simulink model "p1_MPU"  (R2023a)
settings: Solver=FixedStepDiscrete  StartTime=0.0  StopTime=inf  FixedStep=Ts_MPU  RelTol=1e-3  EnableMultiTasking=on
PreLoadFcn:
  | p1_params_new
  | spiDataDefinition
InitFcn:
  | p1_params_new
  | spiDataDefinition
values from neighbouring files (symbols this model uses):
  B = SSest(T,15)+Boffset    [AACplottingcode.m]    (also in Ext_MPCPara.m = SSD.B; IMECE06plottingcode.m = SSest(T,15); If_alpha_tp_observer.m; If_alpha_tp_observer_for_c_code.m)
undefined symbols (not defined in the file or in its folder): DrivetrainLeft, DrivetrainRight, p1data, p1params, Ts_MPU
libraries: simulink x54, raspberrypiBasiclib x8, raspberrypiCommlib x4, embedlinuxNetworklib x2
(part 1 of 2)
settings Model: SimulationMode=external  ExtModeTrigDuration=2  Creator=Audesse  LastModifiedBy=cbeal
settings SolverCC: AlgebraicLoopSolver=TrustRegion  PositivePriorityOrder=on
settings DataIOCC: ReturnWorkspaceOutputs=off  LoggingFileName=MPU_Data.mat
settings OptimizationCC: DefaultUnderspecifiedDataType=single  EnhancedBackFolding=on  PassReuseOutputArgsAs=Individual arguments  MaxStackSize=64  SimCompilerOptimization=on  OptimizeBlockOrder=speed  DifferentSizesBufferReuse=on  OptimizationCustomize=off  EfficientTunableParamExpr=on
settings DebuggingCC: MultiTaskDSMMsg=none  ParameterTunabilityLossMsg=error  UnconnectedInputMsg=warning  UnconnectedOutputMsg=warning  UnconnectedLineMsg=warning
settings HardwareCC: ProdBitPerPointer=32  ProdBitPerSizeT=32  ProdBitPerPtrDiffT=32  ProdLargestAtomicInteger=Long  ProdLargestAtomicFloat=Double  ProdWordSize=32  ProdLongLongMode=on  ProdHWDeviceType=ARM Compatible->ARM Cortex  TargetLargestAtomicInteger=Long  TargetLargestAtomicFloat=Double  TargetLongLongMode=on  TargetIntDivRoundTo=Zero  TargetEndianess=LittleEndian  TargetHWDeviceType=ARM Compatible->ARM Cortex
settings ModelReferenceCC: EnableRefExpFcnMdlSchedulingChecks=on
settings SFSimCC: CustomCodeUndefinedFunction=UseInterfaceOnly
settings RTWCC: Description=Embedded Coder  SystemTargetFile=ert.tlc  HardwareBoard=Raspberry Pi  TLCOptions="-aInlineSetEventsForThisBaseRateFcn=TLC_FALSE -aSuppressMultiTaskScheduler=TLC_FALSE  -aRateBasedStepFcn=0"  TemplateMakefile=ert_default_tmf  Toolchain=GNU GCC Embedded Linux  BuildConfiguration=Faster Runs  IncludeHyperlinkInReport=on  CodeExecutionProfiling=on  CodeProfilingSaveOptions=AllData  CodeProfilingInstrumentation=coarse  DLArmComputeVersion=19.05
settings CodeAppCC: ForceParamTrailComments=on  IgnoreCustomStorageClasses=off  OperatorAnnotations=on  SimulinkDataObjDesc=on  SFDataObjDesc=on  MangleLength=10  InsertBlockDesc=on
settings ERTTargetCC: MatFileLogging=on  SupportNonInlinedSFcns=on  SupportVariableSizeSignals=on  ExtModeTransport=2  ExtModeStaticAlloc=on  ExtModeMexFile=ext_xcp  ExtModeIntrfLevel=Level2 - Open

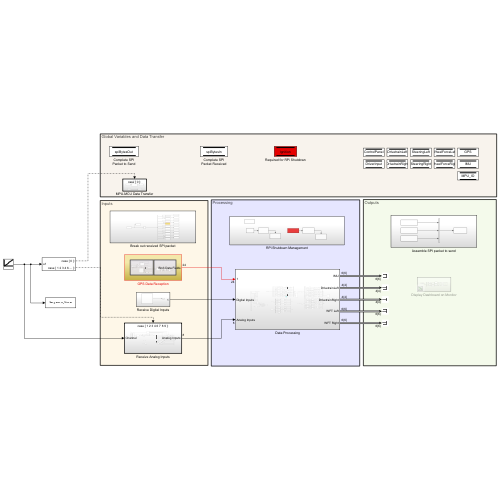
[thumbnail: Simulink's stored preview of the top-level diagram]
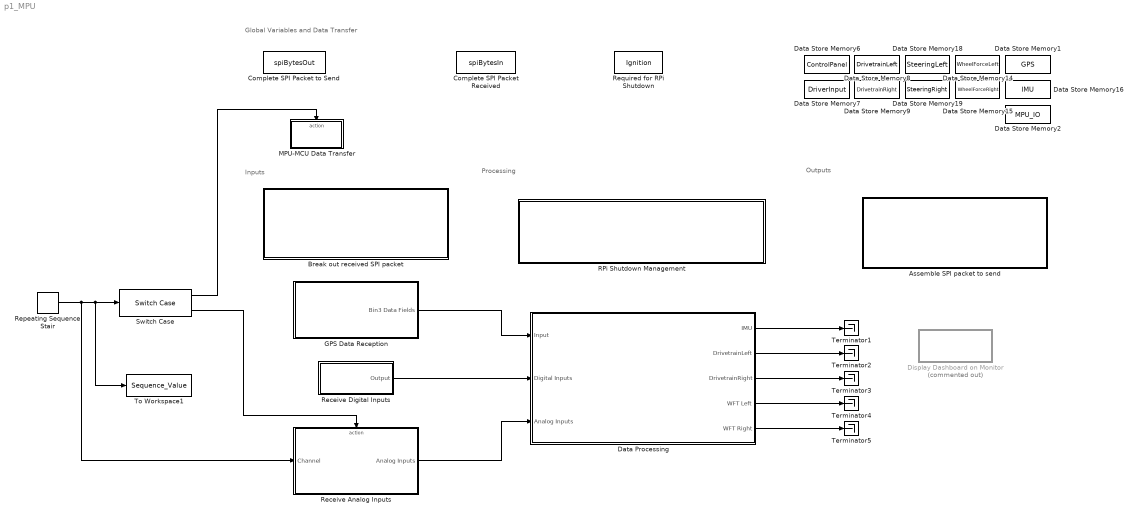
== system p1_MPU ==
  note: Outputs
  note: Processing
  note: Inputs
  note: Global Variables and Data Transfer
  Assemble SPI packet to send : Subsystem
  Break out received SPI packet : Subsystem
  Complete SPI Packet Received : DataStoreMemory  DataStoreName=spiBytesIn  ReadBeforeWriteMsg=warning  WriteAfterWriteMsg=warning  WriteAfterReadMsg=warning  InitialValue=255*ones(p1data.spiBytes,1)  ShowAdditionalParam=off  OutDataTypeStr=uint8
  Complete SPI Packet to Send : DataStoreMemory  DataStoreName=spiBytesOut  ReadBeforeWriteMsg=warning  WriteAfterWriteMsg=warning  WriteAfterReadMsg=warning  InitialValue=zeros(p1data.spiBytes,1)  ShowAdditionalParam=off  OutDataTypeStr=uint8
  Data Processing : Subsystem
  Data Store Memory1 : DataStoreMemory  DataStoreName=GPS  ReadBeforeWriteMsg=warning  WriteAfterWriteMsg=warning  WriteAfterReadMsg=warning  InitialValue=zeros(p1data.gpsBytes,1)  ShowAdditionalParam=off  OutDataTypeStr=uint8
  Data Store Memory14 : DataStoreMemory  DataStoreName=WheelForceLeft  ReadBeforeWriteMsg=warning  WriteAfterWriteMsg=warning  WriteAfterReadMsg=warning  InitialValue=zeros(p1data.wftBytes,1)  ShowAdditionalParam=off  OutDataTypeStr=uint8
  Data Store Memory15 : DataStoreMemory  DataStoreName=WheelForceRight  ReadBeforeWriteMsg=warning  WriteAfterWriteMsg=warning  WriteAfterReadMsg=warning  InitialValue=zeros(p1data.wftBytes,1)  ShowAdditionalParam=off  OutDataTypeStr=uint8
  Data Store Memory16 : DataStoreMemory  DataStoreName=IMU  ReadBeforeWriteMsg=warning  WriteAfterWriteMsg=warning  WriteAfterReadMsg=warning  InitialValue=zeros(p1data.imuBytes,1)  ShowAdditionalParam=off  OutDataTypeStr=uint8
  Data Store Memory18 : DataStoreMemory  DataStoreName=SteeringLeft  ReadBeforeWriteMsg=warning  WriteAfterWriteMsg=warning  WriteAfterReadMsg=warning  InitialValue=zeros(p1data.steeringBytes,1)  ShowAdditionalParam=off  OutDataTypeStr=uint8
  Data Store Memory19 : DataStoreMemory  DataStoreName=SteeringRight  ReadBeforeWriteMsg=warning  WriteAfterWriteMsg=warning  WriteAfterReadMsg=warning  InitialValue=zeros(p1data.steeringBytes,1)  ShowAdditionalParam=off  OutDataTypeStr=uint8
  Data Store Memory2 : DataStoreMemory  DataStoreName=MPU_IO  ReadBeforeWriteMsg=warning  WriteAfterWriteMsg=warning  WriteAfterReadMsg=warning  InitialValue=zeros(p1data.mpuBytes,1)  ShowAdditionalParam=off  OutDataTypeStr=uint8
  Data Store Memory6 : DataStoreMemory  DataStoreName=ControlPanel  ReadBeforeWriteMsg=warning  WriteAfterWriteMsg=warning  WriteAfterReadMsg=warning  InitialValue=zeros(p1data.controlPanelBytes,1)  ShowAdditionalParam=off  OutDataTypeStr=uint8
  Data Store Memory7 : DataStoreMemory  DataStoreName=DriverInput  ReadBeforeWriteMsg=warning  WriteAfterWriteMsg=warning  WriteAfterReadMsg=warning  InitialValue=zeros(p1data.driverInputBytes,1)  ShowAdditionalParam=off  OutDataTypeStr=uint8
  Data Store Memory8 : DataStoreMemory  DataStoreName=DrivetrainLeft  ReadBeforeWriteMsg=warning  WriteAfterWriteMsg=warning  WriteAfterReadMsg=warning  InitialValue=zeros(p1data.drivetrainBytes,1)  ShowAdditionalParam=off  OutDataTypeStr=uint8
  Data Store Memory9 : DataStoreMemory  DataStoreName=DrivetrainRight  ReadBeforeWriteMsg=warning  WriteAfterWriteMsg=warning  WriteAfterReadMsg=warning  InitialValue=zeros(p1data.drivetrainBytes,1)  ShowAdditionalParam=off  OutDataTypeStr=uint8
  Display Dashboard on Monitor : Subsystem  Commented=on
  GPS Data Reception : Subsystem
  MPU-MCU Data Transfer : Subsystem  TreatAsAtomicUnit=on
  RPi Shutdown Management : Subsystem
  Receive Analog Inputs : Subsystem  TreatAsAtomicUnit=on
  Receive Digital Inputs : Subsystem
  Repeating Sequence Stair : simulink/Sources/Repeating Sequence Stair  OutValues=(0:9)'  tsamp=-1  OutMin=[]  OutMax=[]  OutDataTypeStr=uint8  OutputDataTypeScalingMode=uint8  OutDataType=fixdt(0,8)  ConRadixGroup=Best Precision: Vector-wise  OutScaling=2^-12
  Required for RPi Shutdown : DataStoreMemory  DataStoreName=Ignition  ReadBeforeWriteMsg=warning  WriteAfterWriteMsg=warning  WriteAfterReadMsg=warning  ShowAdditionalParam=off  OutDataTypeStr=uint8
  Switch Case : SwitchCase  CaseConditions={[0],[1,2,3,4,6,7,8,9]}  ShowDefaultCase=off
  Terminator{1..5} (5 alike) : Terminator
  To Workspace1 : ToWorkspace  VariableName=Sequence_Value  SampleTime=-1
  wires:
  Data Processing/1(IMU) -> Terminator1/1
  Data Processing/2(DrivetrainLeft) -> Terminator2/1
  Data Processing/3(DrivetrainRight) -> Terminator3/1
  Data Processing/4(WFT Left) -> Terminator4/1
  Data Processing/5(WFT Right) -> Terminator5/1
  Switch Case/1 -> MPU-MCU Data Transfer/Action
  Receive Analog Inputs/1(Analog Inputs) -> Data Processing/3(Analog Inputs)
  Receive Digital Inputs/1(Output) -> Data Processing/2(Digital Inputs)
  GPS Data Reception/1(Bin3 Data Fields) -> Data Processing/1(Input)
  Repeating Sequence Stair/1 -> Switch Case/1, To Workspace1/1, Receive Analog Inputs/1(Channel)
  Switch Case/2 -> Receive Analog Inputs/Action

== system p1_MPU/Assemble SPI packet to send ==
  Data Store Read : DataStoreRead  DataStoreName=GPS  IndexOptions=Index vector (dialog)  Indices=1  OutputSizes=1
  Data Store Read1 : DataStoreRead  DataStoreName=MPU_IO  IndexOptions=Index vector (dialog)  Indices=1  OutputSizes=1
  Data Store Write : DataStoreWrite  DataStoreName=spiBytesOut  IndexOptions=Index vector (dialog)  Indices=1  OutputSizes=1
  Mux : Mux  Inputs=3
  Padding : Constant  Value=zeros(p1data.mpuPadding,1)  OutDataTypeStr=uint8
  wires:
  Mux/1 -> Data Store Write/1
  Padding/1 -> Mux/3
  Data Store Read/1 -> Mux/1
  Data Store Read1/1 -> Mux/2

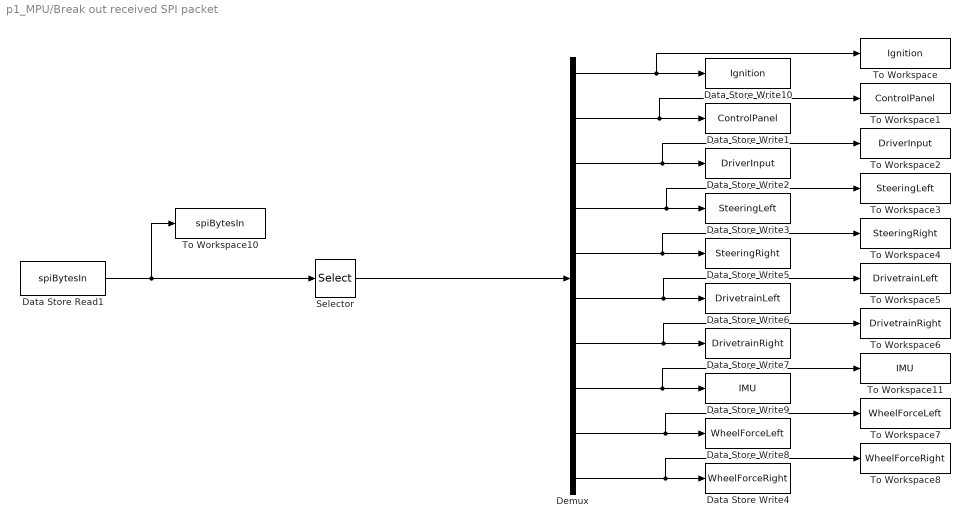
== system p1_MPU/Break out received SPI packet ==
  Data Store Read1 : DataStoreRead  DataStoreName=spiBytesIn  IndexOptions=Index vector (dialog)  Indices=1  OutputSizes=1
  Data Store Write1 : DataStoreWrite  DataStoreName=ControlPanel  IndexOptions=Index vector (dialog)  Indices=1  OutputSizes=1
  Data Store Write10 : DataStoreWrite  DataStoreName=Ignition  IndexOptions=Index vector (dialog)  Indices=1  OutputSizes=1
  Data Store Write2 : DataStoreWrite  DataStoreName=DriverInput  IndexOptions=Index vector (dialog)  Indices=1  OutputSizes=1
  Data Store Write3 : DataStoreWrite  DataStoreName=SteeringLeft  IndexOptions=Index vector (dialog)  Indices=1  OutputSizes=1
  Data Store Write4 : DataStoreWrite  DataStoreName=WheelForceRight  IndexOptions=Index vector (dialog)  Indices=1  OutputSizes=1
  Data Store Write5 : DataStoreWrite  DataStoreName=SteeringRight  IndexOptions=Index vector (dialog)  Indices=1  OutputSizes=1
  Data Store Write6 : DataStoreWrite  DataStoreName=DrivetrainLeft  IndexOptions=Index vector (dialog)  Indices=1  OutputSizes=1
  Data Store Write7 : DataStoreWrite  DataStoreName=DrivetrainRight  IndexOptions=Index vector (dialog)  Indices=1  OutputSizes=1
  Data Store Write8 : DataStoreWrite  DataStoreName=WheelForceLeft  IndexOptions=Index vector (dialog)  Indices=1  OutputSizes=1
  Data Store Write9 : DataStoreWrite  DataStoreName=IMU  IndexOptions=Index vector (dialog)  Indices=1  OutputSizes=1
  Demux : Demux  Outputs=10
  Selector : Selector  InputPortWidth=p1data.spiBytes  IndexOptions=Index vector (dialog)  Indices=[11:225]  OutputSizes=1
  To Workspace : ToWorkspace  VariableName=Ignition  SampleTime=-1
  To Workspace1 : ToWorkspace  VariableName=ControlPanel  SampleTime=-1
  To Workspace10 : ToWorkspace  VariableName=spiBytesIn  SampleTime=-1
      settings: Save2DSignal=2-D array (concatenate along first dimension)
  To Workspace11 : ToWorkspace  VariableName=IMU  SampleTime=-1
  To Workspace2 : ToWorkspace  VariableName=DriverInput  SampleTime=-1
  To Workspace3 : ToWorkspace  VariableName=SteeringLeft  SampleTime=-1
  To Workspace4 : ToWorkspace  VariableName=SteeringRight  SampleTime=-1
  To Workspace5 : ToWorkspace  VariableName=DrivetrainLeft  SampleTime=-1
  To Workspace6 : ToWorkspace  VariableName=DrivetrainRight  SampleTime=-1
  To Workspace7 : ToWorkspace  VariableName=WheelForceLeft  SampleTime=-1
  To Workspace8 : ToWorkspace  VariableName=WheelForceRight  SampleTime=-1
  wires:
  Demux/5 -> Data Store Write5/1, To Workspace4/1
  Demux/1 -> To Workspace/1, Data Store Write10/1
  Demux/9 -> To Workspace7/1, Data Store Write8/1
  Demux/4 -> To Workspace3/1, Data Store Write3/1
  Demux/2 -> Data Store Write1/1, To Workspace1/1
  Demux/6 -> To Workspace5/1, Data Store Write6/1
  Demux/7 -> To Workspace6/1, Data Store Write7/1
  Demux/3 -> To Workspace2/1, Data Store Write2/1
  Demux/10 -> To Workspace8/1, Data Store Write4/1
  Demux/8 -> To Workspace11/1, Data Store Write9/1
  Data Store Read1/1 -> Selector/1, To Workspace10/1
  Selector/1 -> Demux/1

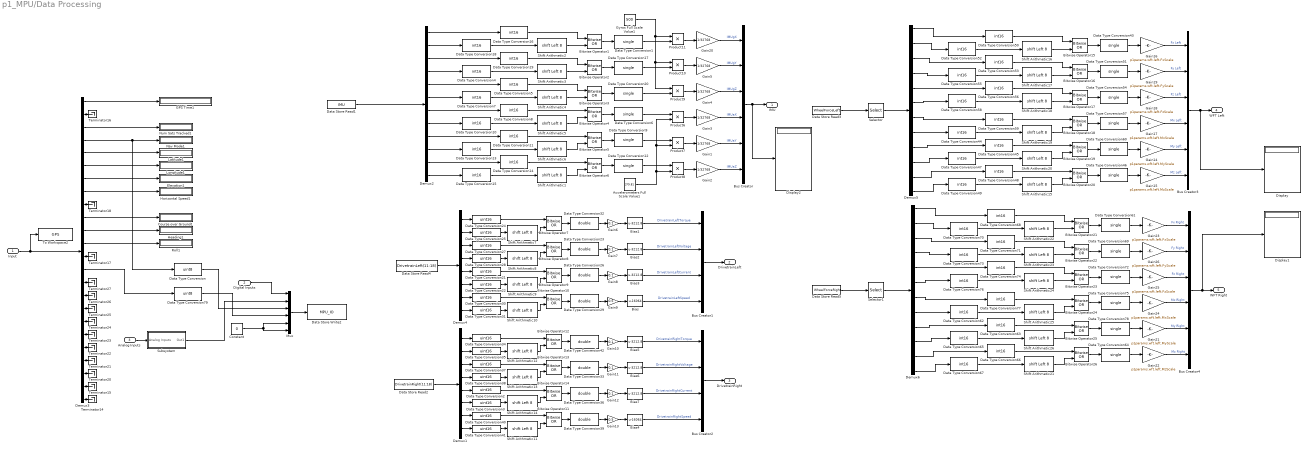
== system p1_MPU/Data Processing ==
  Input : Inport
  Digital Inputs : Inport  Port=2
  Analog Inputs : Inport  Port=3
  Accelerometers Full Scale Value1 : Constant  Value=2*9.81
  Bias : Bias  Bias=-16064  SaturateOnIntegerOverflow=off
  Bias{1..3,5..7} (6 alike) : Bias  Bias=-3212.8  SaturateOnIntegerOverflow=off
  Bias4 : Bias  Bias=-16064  SaturateOnIntegerOverflow=off
  Bitwise Operator{1..26} (26 alike) : simulink/Logic and Bit Operations/Bitwise Operator  logicop=OR  UseBitMask=off  NumInputPorts=2  BitMask=bin2dec('11011001')  BitMaskRealWorld=Stored Integer
  Bus Creator : BusCreator  Inputs=6
  Bus Creator1 : BusCreator  Inputs=4
  Bus Creator2 : BusCreator  Inputs=4
  Bus Creator3 : BusCreator  Inputs=6
  Bus Creator4 : BusCreator  Inputs=6
  Constant : Constant  Value=0  OutDataTypeStr=uint8
  Course over Ground1 : Display
  Data Store Read1 : DataStoreRead  DataStoreName=IMU  IndexOptions=Index vector (dialog)  Indices=1  OutputSizes=1
  Data Store Read2 : DataStoreRead  DataStoreName=DrivetrainRight  DataStoreElements=DrivetrainRight(11:18)  IndexOptions=Index vector (dialog)  Indices=1  OutputSizes=1
  Data Store Read3 : DataStoreRead  DataStoreName=WheelForceLeft  IndexOptions=Index vector (dialog)  Indices=1  OutputSizes=1
  Data Store Read4 : DataStoreRead  DataStoreName=DrivetrainLeft  DataStoreElements=DrivetrainLeft(11:18)  IndexOptions=Index vector (dialog)  Indices=1  OutputSizes=1
  Data Store Read5 : DataStoreRead  DataStoreName=WheelForceRight  IndexOptions=Index vector (dialog)  Indices=1  OutputSizes=1
  Data Store Write2 : DataStoreWrite  DataStoreName=MPU_IO  IndexOptions=Index vector (dialog)  Indices=1  OutputSizes=1
  Data Type Conversion : DataTypeConversion  OutDataTypeStr=uint8  SaturateOnIntegerOverflow=off  RndMeth=Floor
  Data Type Conversion{1,6,9,12,17,20,43,46,51,54,57,60..61,64,69,72,75,78} (18 alike) : DataTypeConversion  OutDataTypeStr=single  SaturateOnIntegerOverflow=off  RndMeth=Floor
  Data Type Conversion{4..5,7..8,10..11,13..16,18..19,44..45,47..50,52..53,55..56,58..59,62..63,65..68,70..71,73..74,76..77} (36 alike) : DataTypeConversion  OutDataTypeStr=int16  ConvertRealWorld=Stored Integer (SI)  SaturateOnIntegerOverflow=off  RndMeth=Floor
  Data Type Conversion{2..3,21..22,24..25,27..28,30..31,34..35,37..38,40..41} (16 alike) : DataTypeConversion  OutDataTypeStr=uint16  SaturateOnIntegerOverflow=off  RndMeth=Floor
  Data Type Conversion{23,26,29,32..33,36,39,42} (8 alike) : DataTypeConversion  OutDataTypeStr=double  SaturateOnIntegerOverflow=off  RndMeth=Floor
  Data Type Conversion79 : DataTypeConversion  OutDataTypeStr=uint8  SaturateOnIntegerOverflow=off  RndMeth=Floor
  Demux1 : Demux  Outputs=8
  Demux2 : Demux  Outputs=12
  Demux3 : Demux  Outputs=24
  Demux4 : Demux  Outputs=8
  Demux5 : Demux  Outputs=12
  Demux6 : Demux  Outputs=12
  Display : Display
  Display1 : Display
  Display2 : Display
  Elevation1 : Display
  GPS Time1 : Display
      settings: Format=long_e
  Gain{1..5,20} (6 alike) : Gain  Gain=1/32768
  Gain{6..8,10..12} (6 alike) : Gain  Gain=0.1  OutDataTypeStr=Inherit: Same as input
  Gain13 : Gain  Gain=0.5  OutDataTypeStr=Inherit: Same as input
  Gain14 : Gain  Gain=p1params.wft.left.MyScale
  Gain15 : Gain  Gain=p1params.wft.left.MzScale
  Gain16 : Gain  Gain=p1params.wft.left.FxScale
  Gain17 : Gain  Gain=p1params.wft.left.MxScale
  Gain18 : Gain  Gain=p1params.wft.left.FzScale
  Gain19 : Gain  Gain=p1params.wft.left.FyScale
  Gain21 : Gain  Gain=p1params.wft.left.MyScale
  Gain22 : Gain  Gain=p1params.wft.left.MzScale
  Gain23 : Gain  Gain=p1params.wft.left.FxScale
  Gain24 : Gain  Gain=p1params.wft.left.MxScale
  Gain25 : Gain  Gain=p1params.wft.left.FzScale
  Gain26 : Gain  Gain=p1params.wft.left.FyScale
  Gain9 : Gain  Gain=0.5  OutDataTypeStr=Inherit: Same as input
  Gyros Full Scale Value1 : Constant  Value=500
  Heading1 : Display
  Horizontal Speed1 : Display
  Latitude1 : Display
  Longitude1 : Display
  Mux : Mux  Inputs=6
  Nav Mode1 : Display
  Num Sats Tracked1 : Display
  Product{6..11} (6 alike) : Product
  Roll1 : Display
  Selector : Selector  InputPortWidth=20  IndexOptions=Index vector (dialog)  Indices=[1:12]  OutputSizes=1
  Selector1 : Selector  InputPortWidth=20  IndexOptions=Index vector (dialog)  Indices=[1:12]  OutputSizes=1
  Shift Arithmetic{1..26} (26 alike) : ArithShift  BitShiftNumber=8  BitShiftDirection=Left
  Subsystem : Subsystem
  Terminator{14..18,20..27} (13 alike) : Terminator
  To Workspace2 : ToWorkspace  VariableName=GPS  SampleTime=-1
      settings: Save2DSignal=2-D array (concatenate along first dimension)
  IMU : Outport
  DrivetrainLeft : Outport  Port=2
  DrivetrainRight : Outport  Port=3
  WFT Left : Outport  Port=4
  WFT Right : Outport  Port=5
  wires:
  Data Store Read1/1 -> Demux2/1
  Data Type Conversion23/1 -> Gain7/1
  Data Type Conversion26/1 -> Gain8/1
  Data Type Conversion32/1 -> Gain6/1
  Demux4/8 -> Data Type Conversion31/1
  Data Type Conversion30/1 -> Bitwise Operator10/1
  Gain6/1 -> Bias1/1
  Data Type Conversion29/1 -> Gain9/1
  Demux4/7 -> Data Type Conversion30/1
  Bitwise Operator10/1 -> Data Type Conversion29/1
  Bitwise Operator7/1 -> Data Type Conversion32/1
  Bitwise Operator9/1 -> Data Type Conversion26/1
  Bitwise Operator8/1 -> Data Type Conversion23/1
  Data Store Read4/1 -> Demux4/1
  Demux4/1 -> Data Type Conversion24/1
  Demux4/2 -> Data Type Conversion25/1
  Demux4/3 -> Data Type Conversion27/1
  Demux4/4 -> Data Type Conversion28/1
  Demux4/5 -> Data Type Conversion21/1
  Demux4/6 -> Data Type Conversion22/1
  Data Type Conversion21/1 -> Bitwise Operator9/1
  Data Type Conversion27/1 -> Bitwise Operator8/1
  Data Type Conversion24/1 -> Bitwise Operator7/1
  Bias1/1 -> Bus Creator1/1  "DrivetrainLeftTorque"
  Gain7/1 -> Bias2/1
  Bias2/1 -> Bus Creator1/2  "DrivetrainLeftVoltage"
  Gain9/1 -> Bias/1
  Bias/1 -> Bus Creator1/4  "DrivetrainLeftSpeed"
  Gain8/1 -> Bias3/1
  Bias3/1 -> Bus Creator1/3  "DrivetrainLeftCurrent"
  Data Type Conversion25/1 -> Shift Arithmetic7/1
  Data Type Conversion31/1 -> Shift Arithmetic10/1
  Data Type Conversion22/1 -> Shift Arithmetic9/1
  Data Type Conversion28/1 -> Shift Arithmetic8/1
  Shift Arithmetic7/1 -> Bitwise Operator7/2
  Shift Arithmetic8/1 -> Bitwise Operator8/2
  Shift Arithmetic9/1 -> Bitwise Operator9/2
  Shift Arithmetic10/1 -> Bitwise Operator10/2
  Shift Arithmetic11/1 -> Bitwise Operator11/2
  Shift Arithmetic14/1 -> Bitwise Operator14/2
  Shift Arithmetic13/1 -> Bitwise Operator13/2
  Shift Arithmetic12/1 -> Bitwise Operator12/2
  Data Type Conversion38/1 -> Shift Arithmetic13/1
  Data Type Conversion3/1 -> Shift Arithmetic14/1
  Data Type Conversion41/1 -> Shift Arithmetic11/1
  Data Type Conversion35/1 -> Shift Arithmetic12/1
  Gain12/1 -> Bias7/1
  Gain13/1 -> Bias4/1
  Gain11/1 -> Bias6/1
  Data Type Conversion34/1 -> Bitwise Operator12/1
  Data Type Conversion37/1 -> Bitwise Operator13/1
  Data Type Conversion2/1 -> Bitwise Operator14/1
  Demux1/6 -> Data Type Conversion3/1
  Demux1/5 -> Data Type Conversion2/1
  Demux1/4 -> Data Type Conversion38/1
  Demux1/3 -> Data Type Conversion37/1
  Demux1/2 -> Data Type Conversion35/1
  Demux1/1 -> Data Type Conversion34/1
  Data Store Read2/1 -> Demux1/1
  Bitwise Operator13/1 -> Data Type Conversion33/1
  Bitwise Operator14/1 -> Data Type Conversion36/1
  Bitwise Operator12/1 -> Data Type Conversion42/1
  Bitwise Operator11/1 -> Data Type Conversion39/1
  Demux1/7 -> Data Type Conversion40/1
  Data Type Conversion39/1 -> Gain13/1
  Gain10/1 -> Bias5/1
  Data Type Conversion40/1 -> Bitwise Operator11/1
  Demux1/8 -> Data Type Conversion41/1
  Data Type Conversion42/1 -> Gain10/1
  Data Type Conversion36/1 -> Gain12/1
  Data Type Conversion33/1 -> Gain11/1
  Bus Creator/1 -> Display2/1, IMU/1
  Bias5/1 -> Bus Creator2/1  "DrivetrainRightTorque"
  Bias6/1 -> Bus Creator2/2  "DrivetrainRightVoltage"
  Bias4/1 -> Bus Creator2/4  "DrivetrainRightSpeed"
  Bias7/1 -> Bus Creator2/3  "DrivetrainRightCurrent"
  Bus Creator1/1 -> DrivetrainLeft/1
  Bus Creator2/1 -> DrivetrainRight/1
  Gyros Full Scale Value1/1 -> Product9/1, Product10/1, Product11/1
  Data Type Conversion10/1 -> Shift Arithmetic5/1
  Data Type Conversion17/1 -> Product10/2
  Demux2/9 -> Data Type Conversion11/1
  Bitwise Operator6/1 -> Data Type Conversion12/1
  Demux2/6 -> Data Type Conversion7/1
  Data Type Conversion20/1 -> Product9/2
  Data Type Conversion13/1 -> Shift Arithmetic6/1
  Product11/1 -> Gain20/1
  Product10/1 -> Gain5/1
  Accelerometers Full Scale Value1/1 -> Product6/2, Product7/2, Product8/2
  Demux2/2 -> Data Type Conversion18/1
  Data Type Conversion6/1 -> Product6/1
  Demux2/1 -> Data Type Conversion16/1
  Bitwise Operator1/1 -> Data Type Conversion1/1
  Data Type Conversion15/1 -> Shift Arithmetic1/1
  Bitwise Operator4/1 -> Data Type Conversion6/1
  Product7/1 -> Gain1/1
  Shift Arithmetic5/1 -> Bitwise Operator4/2
  Product9/1 -> Gain4/1
  Product8/1 -> Gain2/1
  Data Type Conversion19/1 -> Bitwise Operator2/1
  Data Type Conversion9/1 -> Product7/1
  Data Type Conversion4/1 -> Shift Arithmetic3/1
  Data Type Conversion12/1 -> Product8/1
  Shift Arithmetic3/1 -> Bitwise Operator2/2
  Bitwise Operator3/1 -> Data Type Conversion20/1
  Product6/1 -> Gain3/1
  Bitwise Operator2/1 -> Data Type Conversion17/1
  Data Type Conversion1/1 -> Product11/2
  Data Type Conversion7/1 -> Shift Arithmetic4/1
  Shift Arithmetic2/1 -> Bitwise Operator1/2
  Data Type Conversion18/1 -> Shift Arithmetic2/1
  Shift Arithmetic4/1 -> Bitwise Operator3/2
  Demux2/4 -> Data Type Conversion4/1
  Shift Arithmetic6/1 -> Bitwise Operator5/2
  Demux2/10 -> Data Type Conversion13/1
  Bitwise Operator5/1 -> Data Type Conversion9/1
  Demux2/3 -> Data Type Conversion19/1
  Shift Arithmetic1/1 -> Bitwise Operator6/2
  Data Type Conversion16/1 -> Bitwise Operator1/1
  Data Type Conversion5/1 -> Bitwise Operator3/1
  Data Type Conversion14/1 -> Bitwise Operator6/1
  Data Type Conversion8/1 -> Bitwise Operator4/1
  Demux2/5 -> Data Type Conversion5/1
  Demux2/8 -> Data Type Conversion10/1
  Data Type Conversion11/1 -> Bitwise Operator5/1
  Demux2/7 -> Data Type Conversion8/1
  Demux2/12 -> Data Type Conversion15/1
  Demux2/11 -> Data Type Conversion14/1
  Gain2/1 -> Bus Creator/6  "IMUaZ"
  Gain1/1 -> Bus Creator/5  "IMUaY"
  Gain3/1 -> Bus Creator/4  "IMUaX"
  Gain4/1 -> Bus Creator/3  "IMUgZ"
  Gain5/1 -> Bus Creator/2  "IMUgY"
  Gain20/1 -> Bus Creator/1  "IMUgX"
  Demux3/5 -> Latitude1/1
  Demux3/8 -> Horizontal Speed1/1
  Demux3/7 -> Elevation1/1
  Demux3/22 -> Terminator20/1
  Demux3/11 -> Heading1/1
  Demux3/6 -> Longitude1/1
  Demux3/1 -> GPS Time1/1
  Demux3/3 -> Num Sats Tracked1/1
  Demux3/21 -> Terminator21/1
  Demux3/20 -> Terminator22/1
  Demux3/9 -> Terminator18/1
  Demux3/15 -> Terminator27/1
  Demux3/19 -> Terminator23/1
  Demux3/24 -> Terminator14/1
  Demux3/10 -> Course over Ground1/1
  Demux3/17 -> Terminator25/1
  Demux3/12 -> Roll1/1
  Demux3/16 -> Terminator26/1
  Demux3/13 -> Terminator17/1
  Demux3/18 -> Terminator24/1
  Demux3/23 -> Terminator15/1
  Demux3/2 -> Terminator16/1
  Input/1 -> Demux3/1, To Workspace2/1
  Shift Arithmetic16/1 -> Bitwise Operator15/2
  Shift Arithmetic17/1 -> Bitwise Operator16/2
  Data Type Conversion45/1 -> Bitwise Operator19/1
  Data Type Conversion56/1 -> Bitwise Operator17/1
  Data Type Conversion57/1 -> Gain17/1
  Bitwise Operator16/1 -> Data Type Conversion51/1
  Shift Arithmetic20/1 -> Bitwise Operator19/2
  Gain14/1 -> Bus Creator3/5  "My Left"
  Demux5/6 -> Data Type Conversion58/1
  Data Type Conversion58/1 -> Shift Arithmetic18/1
  Data Type Conversion55/1 -> Shift Arithmetic17/1
  Data Type Conversion50/1 -> Bitwise Operator15/1
  Demux5/11 -> Data Type Conversion48/1
  Shift Arithmetic19/1 -> Bitwise Operator18/2
  Bitwise Operator18/1 -> Data Type Conversion57/1
  Demux5/8 -> Data Type Conversion44/1
  Demux5/3 -> Data Type Conversion53/1
  Data Type Conversion52/1 -> Shift Arithmetic16/1
  Demux5/4 -> Data Type Conversion55/1
  Gain15/1 -> Bus Creator3/6  "Mz Left"
  Demux5/7 -> Data Type Conversion59/1
  Demux5/10 -> Data Type Conversion47/1
  Bitwise Operator19/1 -> Data Type Conversion60/1
  Data Type Conversion47/1 -> Shift Arithmetic20/1
  Demux5/2 -> Data Type Conversion52/1
  Data Type Conversion51/1 -> Gain19/1
  Data Type Conversion60/1 -> Gain14/1
  Data Type Conversion59/1 -> Bitwise Operator18/1
  Demux5/5 -> Data Type Conversion56/1
  Demux5/1 -> Data Type Conversion50/1
  Gain16/1 -> Bus Creator3/1  "Fx Left"
  Data Type Conversion53/1 -> Bitwise Operator16/1
  Data Type Conversion48/1 -> Bitwise Operator20/1
  Shift Arithmetic15/1 -> Bitwise Operator20/2
  Data Type Conversion49/1 -> Shift Arithmetic15/1
  Gain19/1 -> Bus Creator3/2  "Fy Left"
  Data Type Conversion46/1 -> Gain15/1
  Bitwise Operator17/1 -> Data Type Conversion54/1
  Demux5/12 -> Data Type Conversion49/1
  Bitwise Operator15/1 -> Data Type Conversion43/1
  Shift Arithmetic18/1 -> Bitwise Operator17/2
  Gain17/1 -> Bus Creator3/4  "Mx Left"
  Demux5/9 -> Data Type Conversion45/1
  Data Store Read3/1 -> Selector/1
  Data Type Conversion43/1 -> Gain16/1
  Bus Creator3/1 -> Display/1, WFT Left/1
  Data Type Conversion54/1 -> Gain18/1
  Bitwise Operator20/1 -> Data Type Conversion46/1
  Data Type Conversion44/1 -> Shift Arithmetic19/1
  Gain18/1 -> Bus Creator3/3  "Fz Left"
  Selector/1 -> Demux5/1
  Selector1/1 -> Demux6/1
  Bitwise Operator26/1 -> Data Type Conversion64/1
  Gain23/1 -> Bus Creator4/1  "Fx Right"
  Data Type Conversion62/1 -> Shift Arithmetic25/1
  Data Type Conversion65/1 -> Shift Arithmetic26/1
  Bitwise Operator23/1 -> Data Type Conversion72/1
  Demux6/9 -> Data Type Conversion63/1
  Data Type Conversion77/1 -> Bitwise Operator24/1
  Bus Creator4/1 -> Display1/1, WFT Right/1
  Data Type Conversion72/1 -> Gain25/1
  Gain25/1 -> Bus Creator4/3  "Fz Right"
  Data Type Conversion78/1 -> Gain21/1
  Demux6/12 -> Data Type Conversion67/1
  Data Type Conversion64/1 -> Gain22/1
  Demux6/4 -> Data Type Conversion73/1
  Shift Arithmetic24/1 -> Bitwise Operator23/2
  Gain26/1 -> Bus Creator4/2  "Fy Right"
  Data Type Conversion71/1 -> Bitwise Operator22/1
  Demux6/1 -> Data Type Conversion68/1
  Demux6/6 -> Data Type Conversion76/1
  Shift Arithmetic22/1 -> Bitwise Operator21/2
  Shift Arithmetic23/1 -> Bitwise Operator22/2
  Bitwise Operator24/1 -> Data Type Conversion75/1
  Demux6/5 -> Data Type Conversion74/1
  Data Type Conversion63/1 -> Bitwise Operator25/1
  Data Type Conversion67/1 -> Shift Arithmetic21/1
  Shift Arithmetic21/1 -> Bitwise Operator26/2
  Data Type Conversion73/1 -> Shift Arithmetic23/1
  Gain24/1 -> Bus Creator4/4  "Mx Right"
  Bitwise Operator21/1 -> Data Type Conversion61/1
  Demux6/10 -> Data Type Conversion65/1
  Data Type Conversion69/1 -> Gain26/1
  Data Type Conversion61/1 -> Gain23/1
  Shift Arithmetic26/1 -> Bitwise Operator25/2
  Bitwise Operator25/1 -> Data Type Conversion78/1
  Demux6/3 -> Data Type Conversion71/1
  Data Type Conversion66/1 -> Bitwise Operator26/1
  Data Type Conversion70/1 -> Shift Arithmetic22/1
  Shift Arithmetic25/1 -> Bitwise Operator24/2
  Bitwise Operator22/1 -> Data Type Conversion69/1
  Demux6/11 -> Data Type Conversion66/1
  Demux6/7 -> Data Type Conversion77/1
  Demux6/8 -> Data Type Conversion62/1
  Data Type Conversion68/1 -> Bitwise Operator21/1
  Data Type Conversion74/1 -> Bitwise Operator23/1
  Data Type Conversion75/1 -> Gain24/1
  Demux6/2 -> Data Type Conversion70/1
  Gain22/1 -> Bus Creator4/6  "Mz Right"
  Gain21/1 -> Bus Creator4/5  "My Right"
  Data Type Conversion76/1 -> Shift Arithmetic24/1
  Data Store Read5/1 -> Selector1/1
  Mux/1 -> Data Store Write2/1
  Constant/1 -> Mux/6, Mux/5
  Digital Inputs/1 -> Mux/1
  Subsystem/1(Out1) -> Mux/2
  Analog Inputs/1 -> Subsystem/1(Analog Inputs)
  Demux3/4 -> Data Type Conversion/1, Nav Mode1/1
  Demux3/14 -> Data Type Conversion79/1
  Data Type Conversion/1 -> Mux/3
  Data Type Conversion79/1 -> Mux/4

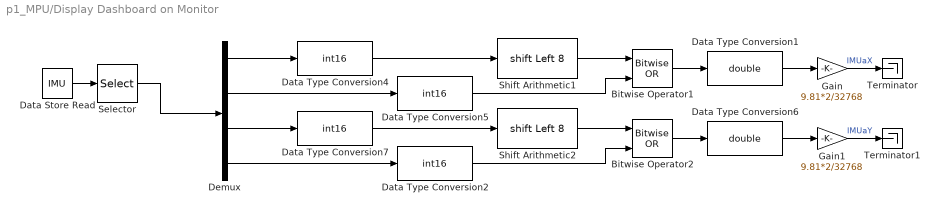
== system p1_MPU/Display Dashboard on Monitor ==
  Bitwise Operator1 : simulink/Logic and Bit Operations/Bitwise Operator  logicop=OR  UseBitMask=off  NumInputPorts=2  BitMask=bin2dec('11011001')  BitMaskRealWorld=Stored Integer
  Bitwise Operator2 : simulink/Logic and Bit Operations/Bitwise Operator  logicop=OR  UseBitMask=off  NumInputPorts=2  BitMask=bin2dec('11011001')  BitMaskRealWorld=Stored Integer
  Data Store Read : DataStoreRead  DataStoreName=IMU  IndexOptions=Index vector (dialog)  Indices=1  OutputSizes=1
  Data Type Conversion1 : DataTypeConversion  OutDataTypeStr=double  SaturateOnIntegerOverflow=off  RndMeth=Floor
  Data Type Conversion{2,4..5,7} (4 alike) : DataTypeConversion  OutDataTypeStr=int16  SaturateOnIntegerOverflow=off  RndMeth=Floor
  Data Type Conversion6 : DataTypeConversion  OutDataTypeStr=double  SaturateOnIntegerOverflow=off  RndMeth=Floor
  Demux : Demux
  Gain : Gain  Gain=9.81*2/32768  OutDataTypeStr=Inherit: Inherit via back propagation
  Gain1 : Gain  Gain=9.81*2/32768  OutDataTypeStr=Inherit: Inherit via back propagation
  Selector : Selector  InputPortWidth=12  IndexOptions=Index vector (dialog)  Indices=[1 2 3 4]  OutputSizes=1
  Shift Arithmetic1 : ArithShift  BitShiftNumber=8  BitShiftDirection=Left
  Shift Arithmetic2 : ArithShift  BitShiftNumber=8  BitShiftDirection=Left
  Terminator : Terminator
  Terminator1 : Terminator
  wires:
  Data Type Conversion7/1 -> Shift Arithmetic2/1
  Demux/2 -> Data Type Conversion5/1
  Shift Arithmetic2/1 -> Bitwise Operator2/1
  Demux/3 -> Data Type Conversion7/1
  Data Type Conversion4/1 -> Shift Arithmetic1/1
  Demux/1 -> Data Type Conversion4/1
  Bitwise Operator2/1 -> Data Type Conversion6/1
  Data Type Conversion6/1 -> Gain1/1
  Bitwise Operator1/1 -> Data Type Conversion1/1
  Data Type Conversion1/1 -> Gain/1
  Data Type Conversion5/1 -> Bitwise Operator1/2
  Shift Arithmetic1/1 -> Bitwise Operator1/1
  Data Type Conversion2/1 -> Bitwise Operator2/2
  Data Store Read/1 -> Selector/1
  Selector/1 -> Demux/1
  Demux/4 -> Data Type Conversion2/1
  Gain1/1 -> Terminator1/1  "IMUaY"
  Gain/1 -> Terminator/1  "IMUaX"

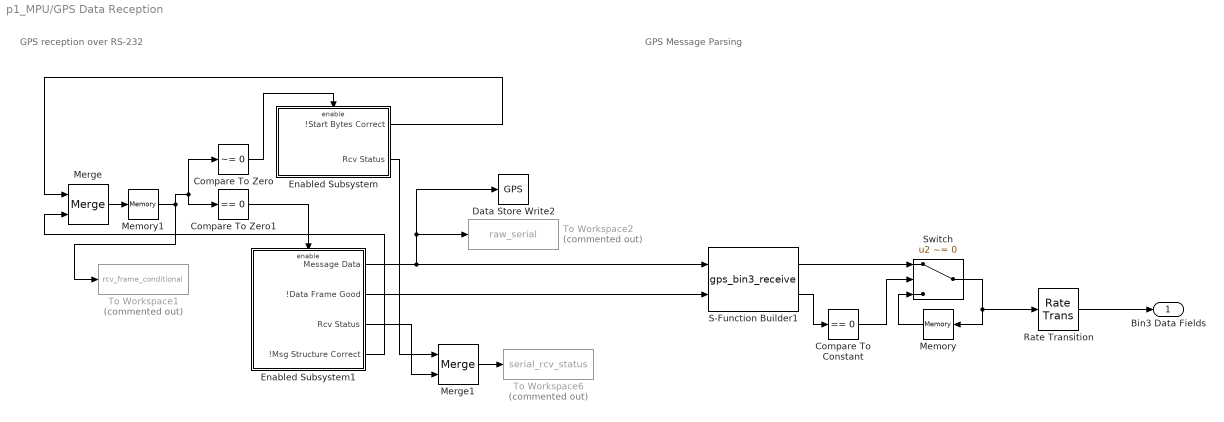
== system p1_MPU/GPS Data Reception ==
  note: GPS Message Parsing
  note: GPS reception over RS-232
  Compare To Constant : simulink/Logic and Bit Operations/Compare To Constant  relop===  const=0  OutDataTypeStr=boolean
  Compare To Zero : simulink/Logic and Bit Operations/Compare To Zero  relop=~=  OutDataTypeStr=boolean
  Compare To Zero1 : simulink/Logic and Bit Operations/Compare To Zero  relop===  OutDataTypeStr=boolean
  Data Store Write2 : DataStoreWrite  DataStoreName=GPS  IndexOptions=Index vector (dialog)  Indices=1  OutputSizes=1
  Enabled Subsystem : Subsystem  TreatAsAtomicUnit=on
  Enabled Subsystem1 : Subsystem  TreatAsAtomicUnit=on
  Memory : Memory  InheritSampleTime=on  LinearizeAsDelay=on
  Memory1 : Memory  InheritSampleTime=on
  Merge : Merge  InitialOutput=0
  Merge1 : Merge  InitialOutput=0
  Rate Transition : RateTransition  OutPortSampleTimeOpt=Inherit
  S-Function Builder1 : S-Function  FunctionName=gps_bin3_receive  SFunctionModules=gps_bin3_receive_wrapper  SFunctionDeploymentMode=off  EnableBusSupport=off  mask(S-Function Builder){}
      mask help: Simulink:masks:SFunctionBuilder_MD
      mask init:
      | val = [[.9  0.75 0.75 1 1 .9 .9 1]',[1 1 0.75 0.75 .9 .9 1 .9]'];try , sys = get_param(gcb,'SfunBuilderFcnName');if isempty(sys), sys = get_param(gcb,'FunctionName'); end,catch, sys = get_param(gcb,'FunctionName'); end
      settings: CopyFcn=set_param(gcbh,'LinkStatus','none')  OpenFcn=sfunctionwizard(gcbh)
      mask Display: plot(val(:,1),val(:,2)),disp(sys),port_label('input',1,'u0'),port_label('input',2,'u1'),port_label('output',1,'y0'),port_label('output',2,'y1')
  Switch : Switch  Criteria=u2 ~= 0  OutDataTypeStr=double  SaturateOnIntegerOverflow=off  InputSameDT=off
  To Workspace1 : ToWorkspace  Commented=on  VariableName=rcv_frame_conditional  SampleTime=-1
      settings: Save2DSignal=2-D array (concatenate along first dimension)
  To Workspace2 : ToWorkspace  Commented=on  VariableName=raw_serial  SampleTime=-1
  To Workspace6 : ToWorkspace  Commented=on  VariableName=serial_rcv_status  SampleTime=-1
      settings: Save2DSignal=2-D array (concatenate along first dimension)
  Bin3 Data Fields : Outport
  wires:
  Enabled Subsystem1/4(!Msg Structure Correct) -> Merge/2
  S-Function Builder1/1 -> Switch/1
  Switch/1 -> Memory/1, Rate Transition/1
  Enabled Subsystem/2(Rcv Status) -> Merge1/1
  Compare To Constant/1 -> Switch/2
  Merge1/1 -> To Workspace6/1
  Enabled Subsystem/1(!Start Bytes Correct) -> Merge/1
  Compare To Zero/1 -> Enabled Subsystem/Enable
  Memory/1 -> Switch/3
  Enabled Subsystem1/2(!Data Frame Good) -> S-Function Builder1/2
  Enabled Subsystem1/3(Rcv Status) -> Merge1/2
  S-Function Builder1/2 -> Compare To Constant/1
  Enabled Subsystem1/1(Message Data) -> Data Store Write2/1, To Workspace2/1, S-Function Builder1/1
  Memory1/1 -> Compare To Zero1/1, Compare To Zero/1, To Workspace1/1
  Merge/1 -> Memory1/1
  Compare To Zero1/1 -> Enabled Subsystem1/Enable
  Rate Transition/1 -> Bin3 Data Fields/1

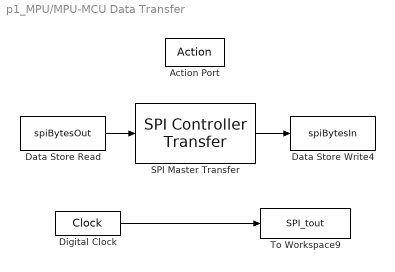
== system p1_MPU/MPU-MCU Data Transfer ==
  Action Port : ActionPort  ActionPortLabel=case [ 0 ]:
  Data Store Read : DataStoreRead  DataStoreName=spiBytesOut  IndexOptions=Index vector (dialog)  Indices=1  OutputSizes=1
  Data Store Write4 : DataStoreWrite  DataStoreName=spiBytesIn  IndexOptions=Index vector (dialog)  Indices=1  OutputSizes=1
  Digital Clock : DigitalClock  SampleTime=Ts_MPU
  SPI Master Transfer : raspberrypiCommlib/SPI Controller Transfer  BoardProperty=Pi 3 Model B+  SSPin=SPI0_CE0  SPIModule=SPI0  Mode=Master  BusSpeed=1000000  Pin=SPI0_CE0  FirstBitToTransfer=Most significant bit (MSB)  ClockMode=2  BlockFunction=Transfer  RegisterAddress=0  OutputDataType=int8  OutputDataLength=1
  To Workspace9 : ToWorkspace  VariableName=SPI_tout  SampleTime=-1
      settings: Save2DSignal=2-D array (concatenate along first dimension)
  wires:
  Data Store Read/1 -> SPI Master Transfer/1
  SPI Master Transfer/1 -> Data Store Write4/1
  Digital Clock/1 -> To Workspace9/1

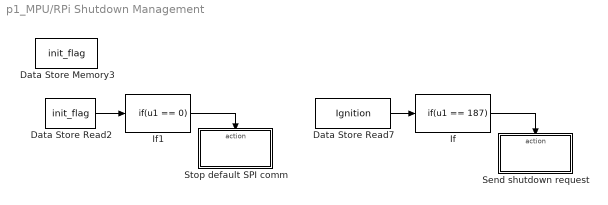
== system p1_MPU/RPi Shutdown Management ==
  Data Store Memory3 : DataStoreMemory  DataStoreName=init_flag  ReadBeforeWriteMsg=warning  WriteAfterWriteMsg=warning  WriteAfterReadMsg=warning  ShowAdditionalParam=off  OutDataTypeStr=uint8
  Data Store Read2 : DataStoreRead  DataStoreName=init_flag  IndexOptions=Index vector (dialog)  Indices=1  OutputSizes=1
  Data Store Read7 : DataStoreRead  DataStoreName=Ignition  IndexOptions=Index vector (dialog)  Indices=1  OutputSizes=1
  If : If  IfExpression=u1 == 187  ShowElse=off
  If1 : If  IfExpression=u1 == 0  ShowElse=off
  Send shutdown request : Subsystem  TreatAsAtomicUnit=on
  Stop default SPI comm : Subsystem  TreatAsAtomicUnit=on
  wires:
  If/1 -> Send shutdown request/Action
  Data Store Read7/1 -> If/1
  If1/1 -> Stop default SPI comm/Action
  Data Store Read2/1 -> If1/1

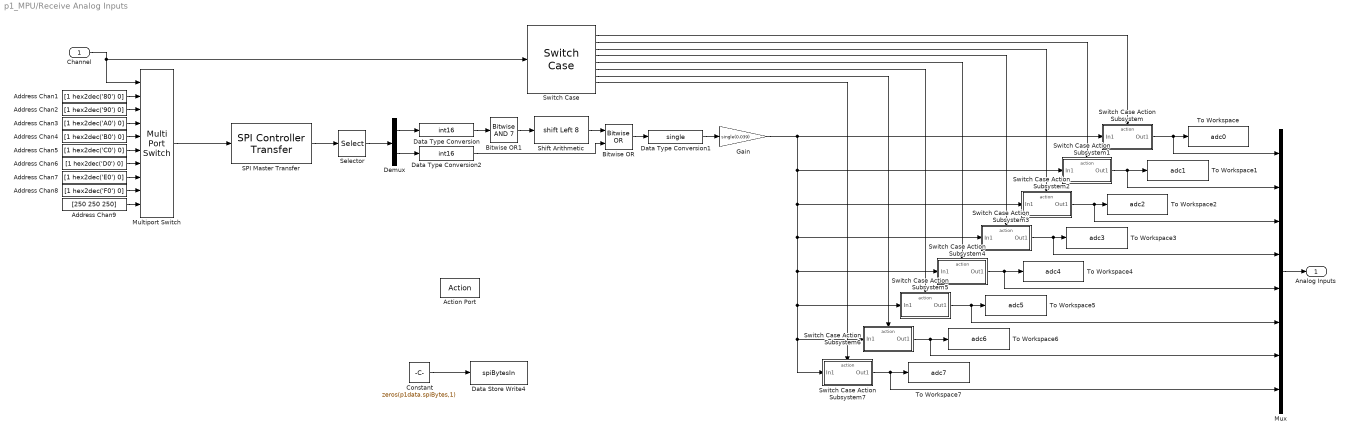
== system p1_MPU/Receive Analog Inputs ==
  Channel : Inport
  Action Port : ActionPort  ActionPortLabel=case [ 1 2 3 4 6 7 8 9 ]:
  Address Chan1 : Constant  Value=[1 hex2dec('80') 0]  OutDataTypeStr=uint8
  Address Chan2 : Constant  Value=[1 hex2dec('90') 0]  OutDataTypeStr=uint8
  Address Chan3 : Constant  Value=[1 hex2dec('A0') 0]  OutDataTypeStr=uint8
  Address Chan4 : Constant  Value=[1 hex2dec('B0') 0]  OutDataTypeStr=uint8
  Address Chan5 : Constant  Value=[1 hex2dec('C0') 0]  OutDataTypeStr=uint8
  Address Chan6 : Constant  Value=[1 hex2dec('D0') 0]  OutDataTypeStr=uint8
  Address Chan7 : Constant  Value=[1 hex2dec('E0') 0]  OutDataTypeStr=uint8
  Address Chan8 : Constant  Value=[1 hex2dec('F0') 0]  OutDataTypeStr=uint8
  Address Chan9 : Constant  Value=[250 250 250]  OutDataTypeStr=uint8
  Bitwise OR : simulink/Logic and Bit Operations/Bitwise Operator  logicop=OR  UseBitMask=off  NumInputPorts=2  BitMask=bin2dec('11011001')  BitMaskRealWorld=Stored Integer
  Bitwise OR1 : simulink/Logic and Bit Operations/Bitwise Operator  logicop=AND  UseBitMask=on  BitMask=7  BitMaskRealWorld=Stored Integer
  Constant : Constant  Value=zeros(p1data.spiBytes,1)  OutDataTypeStr=uint8
  Data Store Write4 : DataStoreWrite  DataStoreName=spiBytesIn  IndexOptions=Index vector (dialog)  Indices=1  OutputSizes=1
  Data Type Conversion : DataTypeConversion  OutDataTypeStr=int16  SaturateOnIntegerOverflow=off  RndMeth=Floor
  Data Type Conversion1 : DataTypeConversion  OutDataTypeStr=single  SaturateOnIntegerOverflow=off  RndMeth=Floor
  Data Type Conversion2 : DataTypeConversion  OutDataTypeStr=int16  SaturateOnIntegerOverflow=off  RndMeth=Floor
  Demux : Demux  Outputs=2
  Gain : Gain  Gain=single(0.039)
  Multiport Switch : MultiPortSwitch  DataPortOrder=Specify indices  Inputs=8  DataPortIndices={1,2,3,4,6,7,8,9}  DataPortForDefault=Additional data port  OutDataTypeStr=uint8  SaturateOnIntegerOverflow=off  InputSameDT=off
  Mux : Mux  Inputs=8
  SPI Master Transfer : raspberrypiCommlib/SPI Controller Transfer  BoardProperty=Pi 4 Model B  SSPin=SPI0_CE1  SPIModule=SPI1  Mode=Master  BusSpeed=1000000  Pin=uint32(0)  FirstBitToTransfer=Most significant bit (MSB)  ClockMode=0  BlockFunction=Transfer  RegisterAddress=0  OutputDataType=int8  OutputDataLength=1
  Selector : Selector  InputPortWidth=3  IndexOptions=Index vector (dialog)  Indices=[2 3]  OutputSizes=1
  Shift Arithmetic : ArithShift  BitShiftNumber=8  BitShiftDirection=Left
  Switch Case : SwitchCase  CaseConditions={1,2,3,4,6,7,8,9}  ShowDefaultCase=off
  Switch Case Action Subsystem : Subsystem  TreatAsAtomicUnit=on
  Switch Case Action Subsystem1 : Subsystem  TreatAsAtomicUnit=on
  Switch Case Action Subsystem2 : Subsystem  TreatAsAtomicUnit=on
  Switch Case Action Subsystem3 : Subsystem  TreatAsAtomicUnit=on
  Switch Case Action Subsystem4 : Subsystem  TreatAsAtomicUnit=on
  Switch Case Action Subsystem5 : Subsystem  TreatAsAtomicUnit=on
  Switch Case Action Subsystem6 : Subsystem  TreatAsAtomicUnit=on
  Switch Case Action Subsystem7 : Subsystem  TreatAsAtomicUnit=on
  To Workspace : ToWorkspace  VariableName=adc0  SampleTime=-1
      settings: Save2DSignal=2-D array (concatenate along first dimension)
  To Workspace1 : ToWorkspace  VariableName=adc1  SampleTime=-1
      settings: Save2DSignal=2-D array (concatenate along first dimension)
  To Workspace2 : ToWorkspace  VariableName=adc2  SampleTime=-1
      settings: Save2DSignal=2-D array (concatenate along first dimension)
  To Workspace3 : ToWorkspace  VariableName=adc3  SampleTime=-1
      settings: Save2DSignal=2-D array (concatenate along first dimension)
  To Workspace4 : ToWorkspace  VariableName=adc4  SampleTime=-1
      settings: Save2DSignal=2-D array (concatenate along first dimension)
  To Workspace5 : ToWorkspace  VariableName=adc5  SampleTime=-1
      settings: Save2DSignal=2-D array (concatenate along first dimension)
  To Workspace6 : ToWorkspace  VariableName=adc6  SampleTime=-1
      settings: Save2DSignal=2-D array (concatenate along first dimension)
  To Workspace7 : ToWorkspace  VariableName=adc7  SampleTime=-1
      settings: Save2DSignal=2-D array (concatenate along first dimension)
  Analog Inputs : Outport
  wires:
  Channel/1 -> Multiport Switch/1, Switch Case/1
  Address Chan8/1 -> Multiport Switch/9
  Switch Case Action Subsystem7/1(Out1) -> Mux/8, To Workspace7/1
  Address Chan4/1 -> Multiport Switch/5
  Switch Case/3 -> Switch Case Action Subsystem2/Action
  Address Chan1/1 -> Multiport Switch/2
  Address Chan5/1 -> Multiport Switch/6
  Demux/1 -> Data Type Conversion/1
  SPI Master Transfer/1 -> Selector/1
  Address Chan6/1 -> Multiport Switch/7
  Switch Case Action Subsystem3/1(Out1) -> Mux/4, To Workspace3/1
  Switch Case/5 -> Switch Case Action Subsystem4/Action
  Switch Case Action Subsystem6/1(Out1) -> Mux/7, To Workspace6/1
  Address Chan7/1 -> Multiport Switch/8
  Address Chan2/1 -> Multiport Switch/3
  Switch Case/6 -> Switch Case Action Subsystem5/Action
  Multiport Switch/1 -> SPI Master Transfer/1
  Switch Case Action Subsystem1/1(Out1) -> Mux/2, To Workspace1/1
  Switch Case/1 -> Switch Case Action Subsystem/Action
  Data Type Conversion1/1 -> Gain/1
  Demux/2 -> Data Type Conversion2/1
  Switch Case Action Subsystem2/1(Out1) -> Mux/3, To Workspace2/1
  Gain/1 -> Switch Case Action Subsystem7/1(In1), Switch Case Action Subsystem6/1(In1), Switch Case Action Subsystem5/1(In1), Switch Case Action Subsystem4/1(In1), Switch Case Action Subsystem3/1(In1), Switch Case Action Subsystem2/1(In1), Switch Case Action Subsystem1/1(In1), Switch Case Action Subsystem/1(In1)
  Address Chan3/1 -> Multiport Switch/4
  Shift Arithmetic/1 -> Bitwise OR/1
  Switch Case/2 -> Switch Case Action Subsystem1/Action
  Selector/1 -> Demux/1
  Bitwise OR1/1 -> Shift Arithmetic/1
  Switch Case/4 -> Switch Case Action Subsystem3/Action
  Data Type Conversion2/1 -> Bitwise OR/2
  Bitwise OR/1 -> Data Type Conversion1/1
  Data Type Conversion/1 -> Bitwise OR1/1
  Switch Case/7 -> Switch Case Action Subsystem6/Action
  Mux/1 -> Analog Inputs/1
  Switch Case Action Subsystem/1(Out1) -> Mux/1, To Workspace/1
  Switch Case/8 -> Switch Case Action Subsystem7/Action
  Switch Case Action Subsystem4/1(Out1) -> Mux/5, To Workspace4/1
  Switch Case Action Subsystem5/1(Out1) -> Mux/6, To Workspace5/1
  Constant/1 -> Data Store Write4/1
  Address Chan9/1 -> Multiport Switch/10

== system p1_MPU/Receive Digital Inputs ==
  Receive DI : Subsystem
  Output : Outport
  wires:
  Receive DI/1(Out1) -> Output/1

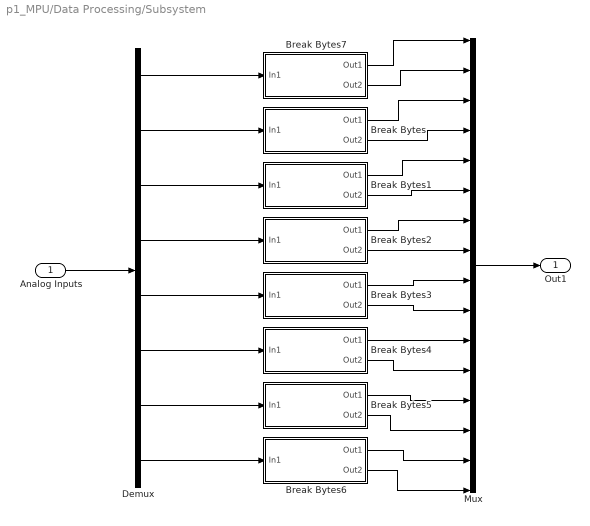
== system p1_MPU/Data Processing/Subsystem ==
  Analog Inputs : Inport
  Break Bytes : Subsystem
  Break Bytes1 : Subsystem
  Break Bytes2 : Subsystem
  Break Bytes3 : Subsystem
  Break Bytes4 : Subsystem
  Break Bytes5 : Subsystem
  Break Bytes6 : Subsystem
  Break Bytes7 : Subsystem
  Demux : Demux  Outputs=8
  Mux : Mux  Inputs=16
  Out1 : Outport
  wires:
  Mux/1 -> Out1/1
  Analog Inputs/1 -> Demux/1
  Demux/1 -> Break Bytes7/1(In1)
  Demux/2 -> Break Bytes/1(In1)
  Demux/3 -> Break Bytes1/1(In1)
  Demux/4 -> Break Bytes2/1(In1)
  Demux/5 -> Break Bytes3/1(In1)
  Demux/6 -> Break Bytes4/1(In1)
  Demux/7 -> Break Bytes5/1(In1)
  Demux/8 -> Break Bytes6/1(In1)
  Break Bytes7/1(Out1) -> Mux/1
  Break Bytes7/2(Out2) -> Mux/2
  Break Bytes/1(Out1) -> Mux/3
  Break Bytes/2(Out2) -> Mux/4
  Break Bytes1/1(Out1) -> Mux/5
  Break Bytes1/2(Out2) -> Mux/6
  Break Bytes2/1(Out1) -> Mux/7
  Break Bytes2/2(Out2) -> Mux/8
  Break Bytes3/2(Out2) -> Mux/10
  Break Bytes3/1(Out1) -> Mux/9
  Break Bytes4/2(Out2) -> Mux/12
  Break Bytes4/1(Out1) -> Mux/11
  Break Bytes5/2(Out2) -> Mux/14
  Break Bytes5/1(Out1) -> Mux/13
  Break Bytes6/2(Out2) -> Mux/16
  Break Bytes6/1(Out1) -> Mux/15

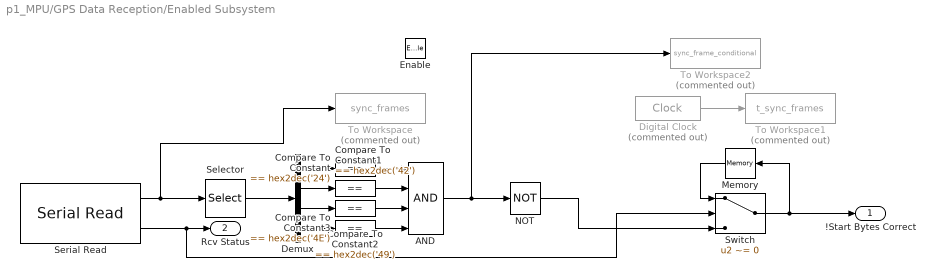
== system p1_MPU/GPS Data Reception/Enabled Subsystem ==
  Enable : EnablePort
  AND : Logic  Inputs=4  IconShape=distinctive  AllPortsSameDT=off  OutDataTypeStr=boolean
  Compare To Constant : simulink/Logic and Bit Operations/Compare To Constant  relop===  const=hex2dec('24')  OutDataTypeStr=boolean
  Compare To Constant1 : simulink/Logic and Bit Operations/Compare To Constant  relop===  const=hex2dec('42')  OutDataTypeStr=boolean
  Compare To Constant2 : simulink/Logic and Bit Operations/Compare To Constant  relop===  const=hex2dec('49')  OutDataTypeStr=boolean
  Compare To Constant3 : simulink/Logic and Bit Operations/Compare To Constant  relop===  const=hex2dec('4E')  OutDataTypeStr=boolean
  Demux : Demux
  Digital Clock : DigitalClock  Commented=on  SampleTime=Ts_MPU
  Memory : Memory  InheritSampleTime=on  LinearizeAsDelay=on
  NOT : Logic  Operator=NOT  IconShape=distinctive  AllPortsSameDT=off  OutDataTypeStr=boolean
  Selector : Selector  InputPortWidth=129  IndexOptions=Index vector (dialog)  Indices=[2:5]  OutputSizes=1
  Serial Read : raspberrypiCommlib/Serial Read  board=Pi 4 Model B  SCIModule_=/dev/serial0  Baudrate_=57600  Parity=None  StopBits_=1  HardwareFlowControl=None  ByteOrder=LittleEndian  DataLength=129  DataType=uint8  OutputStatus=on  SampleTime=p1params.gps.timeStep  blockPlatform=RaspberryPi
  Switch : Switch  Criteria=u2 ~= 0  OutDataTypeStr=double  SaturateOnIntegerOverflow=off  InputSameDT=off
  To Workspace : ToWorkspace  Commented=on  VariableName=sync_frames  SampleTime=-1
  To Workspace1 : ToWorkspace  Commented=on  VariableName=t_sync_frames  SampleTime=-1
      settings: Save2DSignal=2-D array (concatenate along first dimension)
  To Workspace2 : ToWorkspace  Commented=on  VariableName=sync_frame_conditional  SampleTime=-1
      settings: Save2DSignal=2-D array (concatenate along first dimension)
  !Start Bytes Correct : Outport
  Rcv Status : Outport  Port=2
  wires:
  NOT/1 -> Switch/3
  Selector/1 -> Demux/1
  Compare To Constant2/1 -> AND/3
  Demux/1 -> Compare To Constant/1
  Compare To Constant3/1 -> AND/4
  Compare To Constant1/1 -> AND/2
  Serial Read/2 -> Switch/2, Rcv Status/1
  AND/1 -> To Workspace2/1, NOT/1
  Demux/4 -> Compare To Constant3/1
  Compare To Constant/1 -> AND/1
  Demux/2 -> Compare To Constant1/1
  Serial Read/1 -> To Workspace/1, Selector/1
  Demux/3 -> Compare To Constant2/1
  Digital Clock/1 -> To Workspace1/1
  Memory/1 -> Switch/1
  Switch/1 -> !Start Bytes Correct/1, Memory/1

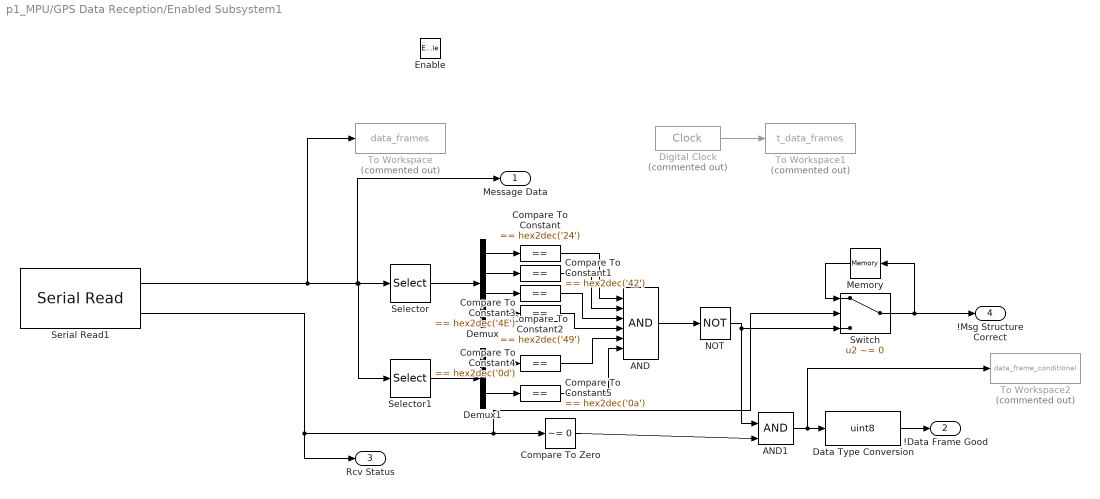
== system p1_MPU/GPS Data Reception/Enabled Subsystem1 ==
  Enable : EnablePort
  AND : Logic  Inputs=6  IconShape=distinctive  AllPortsSameDT=off  OutDataTypeStr=boolean
  AND1 : Logic  IconShape=distinctive  AllPortsSameDT=off  OutDataTypeStr=boolean
  Compare To Constant : simulink/Logic and Bit Operations/Compare To Constant  relop===  const=hex2dec('24')  OutDataTypeStr=boolean
  Compare To Constant1 : simulink/Logic and Bit Operations/Compare To Constant  relop===  const=hex2dec('42')  OutDataTypeStr=boolean
  Compare To Constant2 : simulink/Logic and Bit Operations/Compare To Constant  relop===  const=hex2dec('49')  OutDataTypeStr=boolean
  Compare To Constant3 : simulink/Logic and Bit Operations/Compare To Constant  relop===  const=hex2dec('4E')  OutDataTypeStr=boolean
  Compare To Constant4 : simulink/Logic and Bit Operations/Compare To Constant  relop===  const=hex2dec('0d')  OutDataTypeStr=boolean
  Compare To Constant5 : simulink/Logic and Bit Operations/Compare To Constant  relop===  const=hex2dec('0a')  OutDataTypeStr=boolean
  Compare To Zero : simulink/Logic and Bit Operations/Compare To Zero  relop=~=  OutDataTypeStr=boolean
  Data Type Conversion : DataTypeConversion  OutDataTypeStr=uint8  SaturateOnIntegerOverflow=off  RndMeth=Floor
  Demux : Demux
  Demux1 : Demux  Outputs=2
  Digital Clock : DigitalClock  Commented=on  SampleTime=Ts_MPU
  Memory : Memory  InheritSampleTime=on  LinearizeAsDelay=on
  NOT : Logic  Operator=NOT  IconShape=distinctive  AllPortsSameDT=off  OutDataTypeStr=boolean
  Selector : Selector  InputPortWidth=128  IndexOptions=Index vector (dialog)  Indices=[1:4]  OutputSizes=1
  Selector1 : Selector  InputPortWidth=128  IndexOptions=Index vector (dialog)  Indices=[127:128]  OutputSizes=1
  Serial Read1 : raspberrypiCommlib/Serial Read  board=Pi 4 Model B  SCIModule_=/dev/serial0  Baudrate_=57600  Parity=None  StopBits_=1  HardwareFlowControl=None  ByteOrder=LittleEndian  DataLength=128  DataType=uint8  OutputStatus=on  SampleTime=p1params.gps.timeStep  blockPlatform=RaspberryPi
  Switch : Switch  Criteria=u2 ~= 0  OutDataTypeStr=double  SaturateOnIntegerOverflow=off  InputSameDT=off
  To Workspace : ToWorkspace  Commented=on  VariableName=data_frames  SampleTime=-1
  To Workspace1 : ToWorkspace  Commented=on  VariableName=t_data_frames  SampleTime=-1
      settings: Save2DSignal=2-D array (concatenate along first dimension)
  To Workspace2 : ToWorkspace  Commented=on  VariableName=data_frame_conditional  SampleTime=-1
      settings: Save2DSignal=2-D array (concatenate along first dimension)
  Message Data : Outport
  !Data Frame Good : Outport  Port=2
  Rcv Status : Outport  Port=3
  !Msg Structure Correct : Outport  Port=4
  wires:
  AND1/1 -> To Workspace2/1, Data Type Conversion/1
  Demux1/2 -> Compare To Constant5/1
  Demux1/1 -> Compare To Constant4/1
  Compare To Constant4/1 -> AND/5
  Serial Read1/2 -> Rcv Status/1, Switch/2, Compare To Zero/1
  Demux/4 -> Compare To Constant3/1
  Compare To Constant5/1 -> AND/6
  Digital Clock/1 -> To Workspace1/1
  Selector/1 -> Demux/1
  Compare To Constant2/1 -> AND/3
  Compare To Constant3/1 -> AND/4
  Selector1/1 -> Demux1/1
  AND/1 -> NOT/1
  NOT/1 -> Switch/3, AND1/1
  Compare To Constant/1 -> AND/1
  Demux/1 -> Compare To Constant/1
  Demux/3 -> Compare To Constant2/1
  Compare To Constant1/1 -> AND/2
  Demux/2 -> Compare To Constant1/1
  Serial Read1/1 -> To Workspace/1, Message Data/1, Selector1/1, Selector/1
  Data Type Conversion/1 -> !Data Frame Good/1
  Compare To Zero/1 -> AND1/2
  Switch/1 -> !Msg Structure Correct/1, Memory/1
  Memory/1 -> Switch/1

== system p1_MPU/RPi Shutdown Management/Send shutdown request ==
  Action Port : ActionPort  ActionPortLabel=if(u1 == 187)
  Constant : Constant  Value=187  OutDataTypeStr=uint8
  UDP Send : embedlinuxNetworklib/UDP Send  remoteURL='127.0.0.1'  remotePort=5005  localURL='255.255.255.255'  localPortSource=Automatically determine  localPort=-1  sampletime=-1  blockPlatform=Raspberry Pi  separateLengthPort=0
  wires:
  Constant/1 -> UDP Send/1

== system p1_MPU/RPi Shutdown Management/Stop default SPI comm ==
  Action Port : ActionPort  ActionPortLabel=if(u1 == 0)
  Constant : Constant  OutDataTypeStr=uint8
  Constant1 : Constant  Value=131  OutDataTypeStr=uint8
  Init Flag Write : DataStoreWrite  DataStoreName=init_flag  IndexOptions=Index vector (dialog)  Indices=1  OutputSizes=1
  UDP Send : embedlinuxNetworklib/UDP Send  remoteURL='127.0.0.1'  remotePort=5005  localURL='255.255.255.255'  localPortSource=Automatically determine  localPort=-1  sampletime=-1  blockPlatform=Raspberry Pi  separateLengthPort=0
  wires:
  Constant/1 -> Init Flag Write/1
  Constant1/1 -> UDP Send/1

== system p1_MPU/Receive Analog Inputs/Switch Case Action Subsystem ==
  In1 : Inport
  Action Port : ActionPort  ActionPortLabel=case [ 1 ]:
  Out1 : Outport
  wires:
  In1/1 -> Out1/1

== system p1_MPU/Receive Analog Inputs/Switch Case Action Subsystem1 ==
  In1 : Inport
  Action Port : ActionPort  ActionPortLabel=case [ 2 ]:
  Out1 : Outport
  wires:
  In1/1 -> Out1/1

== system p1_MPU/Receive Analog Inputs/Switch Case Action Subsystem2 ==
  In1 : Inport
  Action Port : ActionPort  ActionPortLabel=case [ 3 ]:
  Out1 : Outport
  wires:
  In1/1 -> Out1/1
